simulink model "KillerWhaleModel"  (R2020b)
settings: Solver=ode15s  StartTime=0.0  StopTime=10.0  MaxStep=0.01  RelTol=1e-3
model workspace: external: MATLAB File KillerWhaleParams.m (data not in the file)
undefined symbols (not defined in the file or in its folder): frontParams, rearParams, standParams, X, Y, Z
libraries: sm_lib x4076, nesl_utility x6
(part 3 of 62)

== system KillerWhaleModel/HeadLinkage/Head_Actuator_1 ==
  Part_10_1_RIGID : Subsystem
  Part_11_1_RIGID : Subsystem
  Part_12_1_RIGID : Subsystem
  Part_13_1_RIGID : Subsystem
  Part_1_1_RIGID : Subsystem
  Part_2_1_RIGID : Subsystem
  Part_3_1_RIGID : Subsystem
  Part_4_1_RIGID : Subsystem
  Part_5_1_RIGID : Subsystem
  Part_6_1_RIGID : Subsystem
  Part_7_1_RIGID : Subsystem
  Part_8_1_RIGID : Subsystem
  Part_9_1_RIGID : Subsystem
  ReferenceFrame : sm_lib/Frames and Transforms/Reference Frame
  Slider1 : sm_lib/Joints/Prismatic Joint  JointMode=Normal  SenseConstraintForce=off  SenseConstraintForceX=off  SenseConstraintForceY=off  SenseConstraintForceZ=off  SenseConstraintTorque=off  SenseConstraintTorqueX=off  SenseConstraintTorqueY=off  SenseConstraintTorqueZ=off  SenseTotalForce=off  SenseTotalForceX=off  SenseTotalForceY=off  SenseTotalForceZ=off  SenseTotalTorque=off  SenseTotalTorqueX=off  SenseTotalTorqueY=off  SenseTotalTorqueZ=off  CompositeWrenchDir=FollowerOnBase  CompositeWrenchFrame=BaseFrame  EquilibriumPosition=0  EquilibriumPositionUnits=m  SpringStiffness=0  SpringStiffnessUnits=N/m  DampingCoefficient=0  DampingCoefficientUnits=N/(m/s)  TorqueActuationMode=ComputedTorque  MotionActuationMode=InputMotion  SensePosition=off  SenseVelocity=off  SenseAcceleration=off  SenseTorqueForce=off  SenseLowerLimitTorqueForce=off  SenseUpperLimitTorqueForce=off  LowerLimitSpecify=off  LowerLimitBound=-1  LowerLimitBoundUnits=m  LowerLimitStiffness=1e6  LowerLimitStiffnessUnits=N/m  LowerLimitDamping=1e3  LowerLimitDampingUnits=N/(m/s)  LowerLimitTransitionRegionWidth=1e-4  LowerLimitTransitionRegionWidthUnits=m  UpperLimitSpecify=off  UpperLimitBound=1  UpperLimitBoundUnits=m  UpperLimitStiffness=1e6  UpperLimitStiffnessUnits=N/m  UpperLimitDamping=1e3  UpperLimitDampingUnits=N/(m/s)  UpperLimitTransitionRegionWidth=1e-4  UpperLimitTransitionRegionWidthUnits=m  PositionTargetSpecify=on  PositionTargetPriority=Low  PositionTargetValue=frontParams.PrismaticJoint(2).Pz.Pos  PositionTargetValueUnits=in  VelocityTargetSpecify=off  VelocityTargetPriority=High  VelocityTargetValue=0  VelocityTargetValueUnits=m/s
  Transform : sm_lib/Frames and Transforms/Rigid Transform  TranslationMethod=Cartesian  TranslationStandardOffset=0  TranslationLengthUnit=in  TranslationStandardAxis=+Z  TranslationCartesianOffset=frontParams.RigidTransform(421).translation  TranslationROffset=0  TranslationROffsetUnits=m  TranslationZOffset=0  TranslationZOffsetUnits=m  TranslationThetaOffset=0  TranslationThetaOffsetUnits=deg  RotationMethod=ArbitraryAxis  RotationAngleUnits=rad  RotationStandardAxis=+Z  RotationAngle=frontParams.RigidTransform(421).angle  RotationArbitraryAxis=frontParams.RigidTransform(421).axis  FollAlignAxisA=+X  BaseAlignAxisA=+Y  FollAlignAxisB=+Y  BaseAlignAxisB=+Z  RotationSequenceAxes=FollowerAxes  RotationSequence=XYX  RotationSequenceAngles=[0 0 0]  RotationSequenceAnglesUnits=deg  RotationMatrix=[1 0 0; 0 1 0; 0 0 1]
  F : PMIOPort  Side=Left
  F1 : PMIOPort  Port=2  Side=Right
  J4 : PMIOPort  Port=3  Side=Right
  connections:
  Part_10_1_RIGID/LConn1 -- Part_5_1_RIGID/LConn2 -- Part_7_1_RIGID/LConn1 -- Part_6_1_RIGID/LConn1 -- Part_4_1_RIGID/LConn1 -- Part_12_1_RIGID/LConn1 -- Part_8_1_RIGID/LConn1
  Part_11_1_RIGID/LConn1 -- Part_2_1_RIGID/LConn1 -- Part_9_1_RIGID/LConn1 -- Part_3_1_RIGID/LConn1 -- Part_13_1_RIGID/LConn1 -- Part_1_1_RIGID/LConn2
  Part_4_1_RIGID/RConn1 -- Slider1/LConn1
  Part_9_1_RIGID/LConn2 -- Slider1/RConn1
  Part_10_1_RIGID/LConn2 -- F/RConn1
  Part_1_1_RIGID/LConn1 -- F1/RConn1
  Part_5_1_RIGID/LConn1 -- Transform/RConn1
  ReferenceFrame/RConn1 -- Transform/LConn1
  J4/RConn1 -- Slider1/LConn2

== system KillerWhaleModel/HeadLinkage/Neck_Actuator_1 ==
  Part_14_1_RIGID : Subsystem
  Part_15_1_RIGID : Subsystem
  Part_16_1_RIGID : Subsystem
  Part_17_1_RIGID : Subsystem
  Part_18_1_RIGID : Subsystem
  Part_19_1_RIGID : Subsystem
  Part_20_1_RIGID : Subsystem
  Part_21_1_RIGID : Subsystem
  Part_22_1_RIGID : Subsystem
  Part_23_1_RIGID : Subsystem
  Part_24_1_RIGID : Subsystem
  Part_25_1_RIGID : Subsystem
  Part_26_1_RIGID : Subsystem
  ReferenceFrame : sm_lib/Frames and Transforms/Reference Frame
  Slider1 : sm_lib/Joints/Prismatic Joint  JointMode=Normal  SenseConstraintForce=off  SenseConstraintForceX=off  SenseConstraintForceY=off  SenseConstraintForceZ=off  SenseConstraintTorque=off  SenseConstraintTorqueX=off  SenseConstraintTorqueY=off  SenseConstraintTorqueZ=off  SenseTotalForce=off  SenseTotalForceX=off  SenseTotalForceY=off  SenseTotalForceZ=off  SenseTotalTorque=off  SenseTotalTorqueX=off  SenseTotalTorqueY=off  SenseTotalTorqueZ=off  CompositeWrenchDir=FollowerOnBase  CompositeWrenchFrame=BaseFrame  EquilibriumPosition=0  EquilibriumPositionUnits=m  SpringStiffness=0  SpringStiffnessUnits=N/m  DampingCoefficient=0  DampingCoefficientUnits=N/(m/s)  TorqueActuationMode=ComputedTorque  MotionActuationMode=InputMotion  SensePosition=off  SenseVelocity=off  SenseAcceleration=off  SenseTorqueForce=off  SenseLowerLimitTorqueForce=off  SenseUpperLimitTorqueForce=off  LowerLimitSpecify=off  LowerLimitBound=-1  LowerLimitBoundUnits=m  LowerLimitStiffness=1e6  LowerLimitStiffnessUnits=N/m  LowerLimitDamping=1e3  LowerLimitDampingUnits=N/(m/s)  LowerLimitTransitionRegionWidth=1e-4  LowerLimitTransitionRegionWidthUnits=m  UpperLimitSpecify=off  UpperLimitBound=1  UpperLimitBoundUnits=m  UpperLimitStiffness=1e6  UpperLimitStiffnessUnits=N/m  UpperLimitDamping=1e3  UpperLimitDampingUnits=N/(m/s)  UpperLimitTransitionRegionWidth=1e-4  UpperLimitTransitionRegionWidthUnits=m  PositionTargetSpecify=on  PositionTargetPriority=Low  PositionTargetValue=frontParams.PrismaticJoint(1).Pz.Pos  PositionTargetValueUnits=in  VelocityTargetSpecify=off  VelocityTargetPriority=High  VelocityTargetValue=0  VelocityTargetValueUnits=m/s
  Transform : sm_lib/Frames and Transforms/Rigid Transform  TranslationMethod=Cartesian  TranslationStandardOffset=0  TranslationLengthUnit=in  TranslationStandardAxis=+Z  TranslationCartesianOffset=frontParams.RigidTransform(420).translation  TranslationROffset=0  TranslationROffsetUnits=m  TranslationZOffset=0  TranslationZOffsetUnits=m  TranslationThetaOffset=0  TranslationThetaOffsetUnits=deg  RotationMethod=ArbitraryAxis  RotationAngleUnits=rad  RotationStandardAxis=+Z  RotationAngle=frontParams.RigidTransform(420).angle  RotationArbitraryAxis=frontParams.RigidTransform(420).axis  FollAlignAxisA=+X  BaseAlignAxisA=+Y  FollAlignAxisB=+Y  BaseAlignAxisB=+Z  RotationSequenceAxes=FollowerAxes  RotationSequence=XYX  RotationSequenceAngles=[0 0 0]  RotationSequenceAnglesUnits=deg  RotationMatrix=[1 0 0; 0 1 0; 0 0 1]
  F : PMIOPort  Side=Left
  J3 : PMIOPort  Port=2  Side=Left
  F1 : PMIOPort  Port=3  Side=Right
  connections:
  Part_14_1_RIGID/LConn1 -- Part_16_1_RIGID/LConn1 -- Part_25_1_RIGID/LConn1 -- Part_23_1_RIGID/LConn2 -- Part_26_1_RIGID/LConn2 -- Part_15_1_RIGID/LConn1
  Part_17_1_RIGID/LConn1 -- Part_21_1_RIGID/LConn1 -- Part_22_1_RIGID/LConn1 -- Part_20_1_RIGID/LConn1 -- Part_19_1_RIGID/LConn1 -- Part_24_1_RIGID/LConn1 -- Part_18_1_RIGID/LConn2
  Part_17_1_RIGID/RConn1 -- Slider1/LConn1
  Part_26_1_RIGID/LConn1 -- Slider1/RConn1
  Part_23_1_RIGID/LConn1 -- F/RConn1
  Part_17_1_RIGID/LConn2 -- F1/RConn1
  Part_18_1_RIGID/LConn1 -- Transform/RConn1
  ReferenceFrame/RConn1 -- Transform/LConn1
  J3/RConn1 -- Slider1/LConn2

== system KillerWhaleModel/RearLinkage/Tail_Actuator_1_1 ==
  Part_40_1_RIGID : Subsystem
  Part_41_1_RIGID : Subsystem
  Part_42_1_RIGID : Subsystem
  Part_43_1_RIGID : Subsystem
  Part_44_1_RIGID : Subsystem
  Part_45_1_RIGID : Subsystem
  Part_46_1_RIGID : Subsystem
  Part_47_1_RIGID : Subsystem
  Part_48_1_RIGID : Subsystem
  Part_49_1_RIGID : Subsystem
  Part_50_1_RIGID : Subsystem
  Part_51_1_RIGID : Subsystem
  Part_52_1_RIGID : Subsystem
  ReferenceFrame : sm_lib/Frames and Transforms/Reference Frame
  Slider1 : sm_lib/Joints/Prismatic Joint  JointMode=Normal  SenseConstraintForce=off  SenseConstraintForceX=off  SenseConstraintForceY=off  SenseConstraintForceZ=off  SenseConstraintTorque=off  SenseConstraintTorqueX=off  SenseConstraintTorqueY=off  SenseConstraintTorqueZ=off  SenseTotalForce=off  SenseTotalForceX=off  SenseTotalForceY=off  SenseTotalForceZ=off  SenseTotalTorque=off  SenseTotalTorqueX=off  SenseTotalTorqueY=off  SenseTotalTorqueZ=off  CompositeWrenchDir=FollowerOnBase  CompositeWrenchFrame=BaseFrame  EquilibriumPosition=0  EquilibriumPositionUnits=m  SpringStiffness=0  SpringStiffnessUnits=N/m  DampingCoefficient=0  DampingCoefficientUnits=N/(m/s)  TorqueActuationMode=ComputedTorque  MotionActuationMode=InputMotion  SensePosition=off  SenseVelocity=off  SenseAcceleration=off  SenseTorqueForce=off  SenseLowerLimitTorqueForce=off  SenseUpperLimitTorqueForce=off  LowerLimitSpecify=off  LowerLimitBound=-1  LowerLimitBoundUnits=m  LowerLimitStiffness=1e6  LowerLimitStiffnessUnits=N/m  LowerLimitDamping=1e3  LowerLimitDampingUnits=N/(m/s)  LowerLimitTransitionRegionWidth=1e-4  LowerLimitTransitionRegionWidthUnits=m  UpperLimitSpecify=off  UpperLimitBound=1  UpperLimitBoundUnits=m  UpperLimitStiffness=1e6  UpperLimitStiffnessUnits=N/m  UpperLimitDamping=1e3  UpperLimitDampingUnits=N/(m/s)  UpperLimitTransitionRegionWidth=1e-4  UpperLimitTransitionRegionWidthUnits=m  PositionTargetSpecify=on  PositionTargetPriority=Low  PositionTargetValue=rearParams.PrismaticJoint(1).Pz.Pos  PositionTargetValueUnits=in  VelocityTargetSpecify=off  VelocityTargetPriority=High  VelocityTargetValue=0  VelocityTargetValueUnits=m/s
  Transform : sm_lib/Frames and Transforms/Rigid Transform  TranslationMethod=Cartesian  TranslationStandardOffset=0  TranslationLengthUnit=in  TranslationStandardAxis=+Z  TranslationCartesianOffset=rearParams.RigidTransform(787).translation  TranslationROffset=0  TranslationROffsetUnits=m  TranslationZOffset=0  TranslationZOffsetUnits=m  TranslationThetaOffset=0  TranslationThetaOffsetUnits=deg  RotationMethod=ArbitraryAxis  RotationAngleUnits=rad  RotationStandardAxis=+Z  RotationAngle=rearParams.RigidTransform(787).angle  RotationArbitraryAxis=rearParams.RigidTransform(787).axis  FollAlignAxisA=+X  BaseAlignAxisA=+Y  FollAlignAxisB=+Y  BaseAlignAxisB=+Z  RotationSequenceAxes=FollowerAxes  RotationSequence=XYX  RotationSequenceAngles=[0 0 0]  RotationSequenceAnglesUnits=deg  RotationMatrix=[1 0 0; 0 1 0; 0 0 1]
  J2 : PMIOPort  Side=Left
  F1 : PMIOPort  Port=2  Side=Right
  F : PMIOPort  Port=3  Side=Right
  connections:
  Part_41_1_RIGID/LConn1 -- Part_42_1_RIGID/LConn1 -- Part_52_1_RIGID/LConn2 -- Part_40_1_RIGID/LConn1 -- Part_49_1_RIGID/LConn1 -- Part_51_1_RIGID/LConn1
  Part_44_1_RIGID/LConn2 -- Part_43_1_RIGID/LConn1 -- Part_47_1_RIGID/LConn1 -- Part_48_1_RIGID/LConn1 -- Part_46_1_RIGID/LConn1 -- Part_45_1_RIGID/LConn1 -- Part_50_1_RIGID/LConn1
  Part_43_1_RIGID/RConn1 -- Slider1/LConn1
  Part_52_1_RIGID/LConn1 -- Slider1/RConn1
  Part_43_1_RIGID/LConn2 -- F/RConn1
  Part_40_1_RIGID/LConn2 -- F1/RConn1
  Part_44_1_RIGID/LConn1 -- Transform/RConn1
  ReferenceFrame/RConn1 -- Transform/LConn1
  J2/RConn1 -- Slider1/LConn2

== system KillerWhaleModel/RearLinkage/Tail_Actuator_2_1 ==
  Part_27_1_RIGID : Subsystem
  Part_28_1_RIGID : Subsystem
  Part_29_1_RIGID : Subsystem
  Part_30_1_RIGID : Subsystem
  Part_31_1_RIGID : Subsystem
  Part_32_1_RIGID : Subsystem
  Part_33_1_RIGID : Subsystem
  Part_34_1_RIGID : Subsystem
  Part_35_1_RIGID : Subsystem
  Part_36_1_RIGID : Subsystem
  Part_37_1_RIGID : Subsystem
  Part_38_1_RIGID : Subsystem
  Part_39_1_RIGID : Subsystem
  ReferenceFrame : sm_lib/Frames and Transforms/Reference Frame
  Slider1 : sm_lib/Joints/Prismatic Joint  JointMode=Normal  SenseConstraintForce=off  SenseConstraintForceX=off  SenseConstraintForceY=off  SenseConstraintForceZ=off  SenseConstraintTorque=off  SenseConstraintTorqueX=off  SenseConstraintTorqueY=off  SenseConstraintTorqueZ=off  SenseTotalForce=off  SenseTotalForceX=off  SenseTotalForceY=off  SenseTotalForceZ=off  SenseTotalTorque=off  SenseTotalTorqueX=off  SenseTotalTorqueY=off  SenseTotalTorqueZ=off  CompositeWrenchDir=FollowerOnBase  CompositeWrenchFrame=BaseFrame  EquilibriumPosition=0  EquilibriumPositionUnits=m  SpringStiffness=0  SpringStiffnessUnits=N/m  DampingCoefficient=0  DampingCoefficientUnits=N/(m/s)  TorqueActuationMode=ComputedTorque  MotionActuationMode=InputMotion  SensePosition=off  SenseVelocity=off  SenseAcceleration=off  SenseTorqueForce=off  SenseLowerLimitTorqueForce=off  SenseUpperLimitTorqueForce=off  LowerLimitSpecify=off  LowerLimitBound=-1  LowerLimitBoundUnits=m  LowerLimitStiffness=1e6  LowerLimitStiffnessUnits=N/m  LowerLimitDamping=1e3  LowerLimitDampingUnits=N/(m/s)  LowerLimitTransitionRegionWidth=1e-4  LowerLimitTransitionRegionWidthUnits=m  UpperLimitSpecify=off  UpperLimitBound=1  UpperLimitBoundUnits=m  UpperLimitStiffness=1e6  UpperLimitStiffnessUnits=N/m  UpperLimitDamping=1e3  UpperLimitDampingUnits=N/(m/s)  UpperLimitTransitionRegionWidth=1e-4  UpperLimitTransitionRegionWidthUnits=m  PositionTargetSpecify=on  PositionTargetPriority=Low  PositionTargetValue=rearParams.PrismaticJoint(2).Pz.Pos  PositionTargetValueUnits=in  VelocityTargetSpecify=off  VelocityTargetPriority=High  VelocityTargetValue=0  VelocityTargetValueUnits=m/s
  Transform : sm_lib/Frames and Transforms/Rigid Transform  TranslationMethod=Cartesian  TranslationStandardOffset=0  TranslationLengthUnit=in  TranslationStandardAxis=+Z  TranslationCartesianOffset=rearParams.RigidTransform(788).translation  TranslationROffset=0  TranslationROffsetUnits=m  TranslationZOffset=0  TranslationZOffsetUnits=m  TranslationThetaOffset=0  TranslationThetaOffsetUnits=deg  RotationMethod=ArbitraryAxis  RotationAngleUnits=rad  RotationStandardAxis=+Z  RotationAngle=rearParams.RigidTransform(788).angle  RotationArbitraryAxis=rearParams.RigidTransform(788).axis  FollAlignAxisA=+X  BaseAlignAxisA=+Y  FollAlignAxisB=+Y  BaseAlignAxisB=+Z  RotationSequenceAxes=FollowerAxes  RotationSequence=XYX  RotationSequenceAngles=[0 0 0]  RotationSequenceAnglesUnits=deg  RotationMatrix=[1 0 0; 0 1 0; 0 0 1]
  J1 : PMIOPort  Side=Left
  F1 : PMIOPort  Port=2  Side=Right
  F : PMIOPort  Port=3  Side=Right
  connections:
  Part_30_1_RIGID/LConn2 -- Part_29_1_RIGID/LConn1 -- Part_33_1_RIGID/LConn1 -- Part_34_1_RIGID/LConn1 -- Part_32_1_RIGID/LConn1 -- Part_31_1_RIGID/LConn1 -- Part_36_1_RIGID/LConn1
  Part_28_1_RIGID/LConn1 -- Part_38_1_RIGID/LConn2 -- Part_39_1_RIGID/LConn2 -- Part_27_1_RIGID/LConn1 -- Part_35_1_RIGID/LConn1 -- Part_37_1_RIGID/LConn1
  Part_29_1_RIGID/RConn1 -- Slider1/LConn1
  Part_38_1_RIGID/LConn1 -- Slider1/RConn1
  Part_29_1_RIGID/LConn2 -- F/RConn1
  Part_39_1_RIGID/LConn1 -- F1/RConn1
  Part_30_1_RIGID/LConn1 -- Transform/RConn1
  ReferenceFrame/RConn1 -- Transform/LConn1
  J1/RConn1 -- Slider1/LConn2
